simulink model "network_sim"  (R2021b)
settings: Solver=VariableStepAuto  StartTime=0.0  StopTime=tstop  RelTol=1e-3
values from neighbouring files (symbols this model uses):
  Anew = (kron(I,A))    [lureconsensus.m]    (also in network_build.m = (kron(eye(4),A)))
  Bnew = (kron(I,B))    [lureconsensus.m]    (also in network_build.m = (kron(eye(4),B)))
  Knew = (kron(Lap,K))    [lureconsensus.m]    (also in network_build.m)
  x0 = rand(12,1)    [lureconsensus.m]    (also in network_build.m)
settings Model: Creator=mct6  LastModifiedBy=sharmin

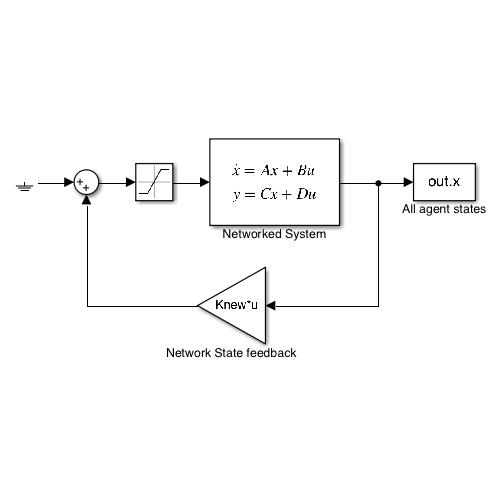
[thumbnail: Simulink's stored preview of the top-level diagram]
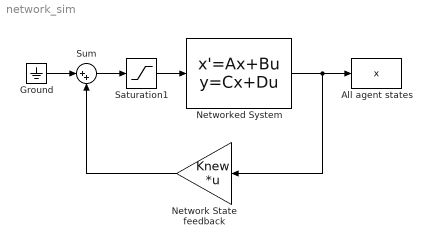
== system network_sim ==
  All agent states : ToWorkspace  VariableName=x  SaveFormat=Structure With Time  SampleTime=-1
  Ground : Ground
  Network State feedback : Gain  Gain=Knew  Multiplication=Matrix(K*u)
  Networked System : StateSpace  A=Anew  B=Bnew  C=eye(12)  D=zeros(12,4)  InitialCondition=x0
  Saturation1 : Saturate
  Sum : Sum  Inputs=|++
  wires:
  Saturation1/1 -> Networked System/1
  Sum/1 -> Saturation1/1
  Ground/1 -> Sum/1
  Networked System/1 -> All agent states/1, Network State feedback/1
  Network State feedback/1 -> Sum/2
